simulink model "simu_6a"  (R2015a)
settings: Solver=ode45  StartTime=0.0  StopTime=60  RelTol=1e-3
undefined symbols (not defined in the file): sigbuilder_block
settings Model: Creator=Aluno-05  LastModifiedBy=Aluno-05

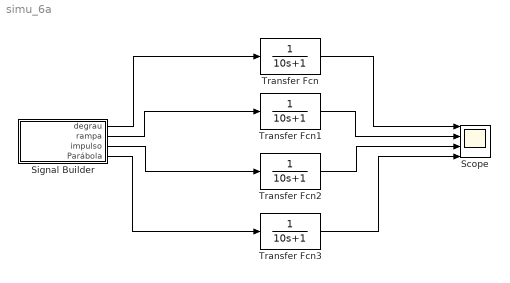
== system simu_6a ==
  Scope : Scope  NumInputPorts=4
      settings: YMin=-1~-1~-1~-1  YMax=1~1~1~1
  Signal Builder : Subsystem  Tag=STV Subsys  LoadFcn=sigbuilder_block('load');  StartFcn=sigbuilder_block('start');  StopFcn=sigbuilder_block('stop');  ClipboardFcn=sigbuilder_block('clipboard');  mask(Sigbuilder block){}
      mask help: Simulink:masks:SigbuilderBlock_MD
      mask init:
      | if ~strcmp(get_param(bdroot(gcbh),'SimulationStatus'),'stopped') tuvar = sigbuilder_block('maskInit'); end
      settings: CopyFcn=sigbuilder_block('copy');  DeleteFcn=sigbuilder_block('delete');  ModelCloseFcn=sigbuilder_block('modelClose');  PreSaveFcn=sigbuilder_block('preSave');  PauseFcn=sigbuilder_block('pause');  ContinueFcn=sigbuilder_block('continue');  NameChangeFcn=sigbuilder_block('namechange');  OpenFcn=sigbuilder_block('open',[437.6 199.2 550.4 400 ]);  CloseFcn=sigbuilder_block('close');
      mask Display: plot(0, 0, 100, 100,[2, 2, 32, 32, 2], [68, 8, 8, 68, 68],[32, 2], [38, 38], [32, 19, 2],[53, 60, 44], [32, 17, 17, 2],[16, 16, 31, 31]);txt = getActiveGroup(gcbh);text(2, 100, txt,'verticalAlignment', 'top');
  Transfer Fcn{,1..3} (4 alike) : TransferFcn  Denominator=[10 1]
  wires:
  Signal Builder/1(degrau) -> Transfer Fcn/1
  Transfer Fcn/1 -> Scope/1
  Signal Builder/2(rampa) -> Transfer Fcn1/1
  Signal Builder/3(impulso) -> Transfer Fcn2/1
  Signal Builder/4(Parábola) -> Transfer Fcn3/1
  Transfer Fcn1/1 -> Scope/2
  Transfer Fcn2/1 -> Scope/3
  Transfer Fcn3/1 -> Scope/4

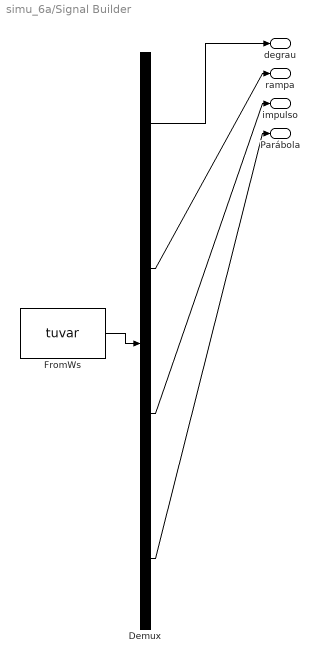
== system simu_6a/Signal Builder ==
  Demux : Demux  Tag=STV Demux
  FromWs : FromWorkspace  Tag=STV FromWs  VariableName=tuvar  SampleTime=0
      SigBuilderData=|
      | common.afterFinalStr = 'Extrapolate'
      | common.sampleTime = 0
      | dataSet.timeRange = [0 60]
      | dataSet.name = 'Group 1'
      | sbobj.Groups.Name = 'Group 1'
      | sbobj.Groups.Signals(1).Name = 'degrau'
      | sbobj.Groups.Signals(1).XData = [0 60]
      | sbobj.Groups.Signals(1).YData = [1 1]
      | sbobj.Groups.Signals(2).Name = 'rampa'
      | sbobj.Groups.Signals(2).XData = [0 0.1 0.2 0.3 0.4 0.5 0.6 0.7 0.8 0.9 1 1.1 ... (601 elements, 1x601)]
      | sbobj.Groups.Signals(2).YData = [0 0.1 0.2 0.3 0.4 0.5 0.6 0.7 0.8 0.9 1 1.1 ... (601 elements, 1x601)]
      | sbobj.Groups.Signals(3).Name = 'impulso'
      | sbobj.Groups.Signals(3).XData = [0 1e-07 1e-07 60]
      | sbobj.Groups.Signals(3).YData = [1 1 0 0]
      | sbobj.Groups.Signals(4).Name = 'Parábola'
      | sbobj.Groups.Signals(4).XData = [0 0.1 0.2 0.3 0.4 0.5 0.6 0.7 0.8 0.9 1 1.1 ... (601 elements, 1x601)]
      | sbobj.Groups.Signals(4).YData = [0 0.01 0.04 0.09 0.16 0.25 0.36 0.49 0.64 0.81 1 1.21 ... (601 elements, 1x601)]
      | sbobj.Groups.TimeRange = [0 60]
  degrau : Outport  Tag=STV Outport
  rampa : Outport  Tag=STV Outport  Port=2
  impulso : Outport  Tag=STV Outport  Port=3
  Parábola : Outport  Tag=STV Outport  Port=4
  wires:
  Demux/1 -> degrau/1
  FromWs/1 -> Demux/1
  Demux/2 -> rampa/1
  Demux/3 -> impulso/1
  Demux/4 -> Parábola/1
